simulink model "project_switchcase"  (R2019a)
settings: Solver=FixedStepDiscrete  StartTime=0.0  StopTime=40  FixedStep=1  RelTol=1e-3
libraries: powerlib_meascontrol x10, simulink x1
settings Model: Creator=admin  LastModifiedBy=admin
settings OptimizationCC: DefaultParameterBehavior=Inlined  EnhancedBackFolding=on  PassReuseOutputArgsAs=Individual arguments  OptimizeBlockOrder=speed  DifferentSizesBufferReuse=on  OptimizationCustomize=off
settings DebuggingCC: ParameterTunabilityLossMsg=error
settings SFSimCC: MATLABDynamicMemAlloc=off
settings RTWCC: SystemTargetFile=ert.tlc  TemplateMakefile=ert_default_tmf  GenerateReport=on  IncludeHyperlinkInReport=on  LaunchReport=on  GenerateTraceInfo=on  GenerateTraceReport=on  GenerateTraceReportSl=on  GenerateTraceReportSf=on  GenerateTraceReportEml=on
settings CodeAppCC: ForceParamTrailComments=on  IgnoreCustomStorageClasses=off  OperatorAnnotations=on  SimulinkDataObjDesc=on  SFDataObjDesc=on  InsertBlockDesc=on
settings ERTTargetCC: TargetLangStandard=C99 (ISO)  GenerateSampleERTMain=on  InlinedParameterPlacement=NonHierarchical  ERTCustomFileTemplate=example_file_process.tlc

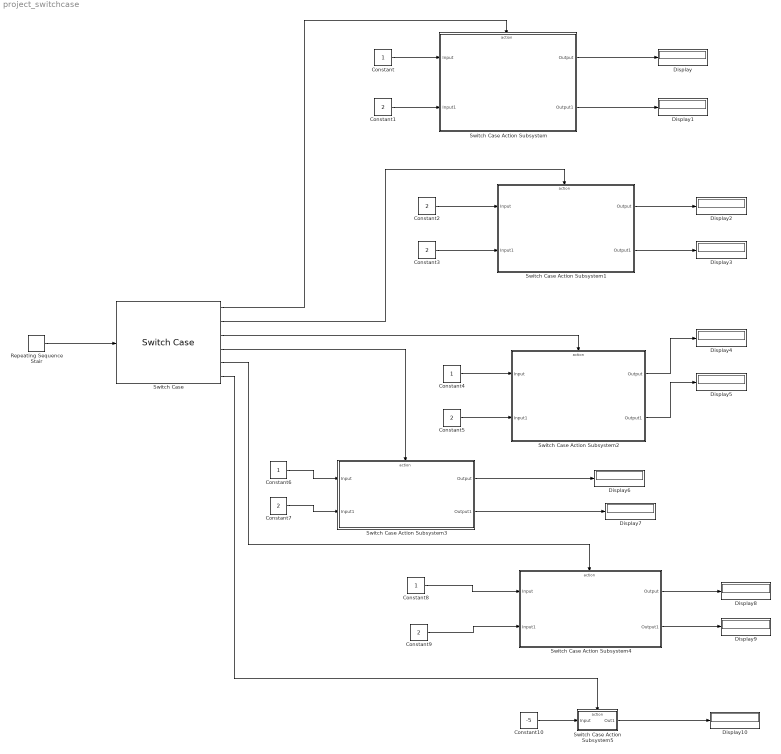
== system project_switchcase ==
  Constant{,4,6,8} (4 alike) : Constant
  Constant{1..3,5,7,9} (6 alike) : Constant  Value=2
  Constant10 : Constant  Value=-5
  Display{,1..10} (11 alike) : Display
  Repeating Sequence Stair : simulink/Sources/Repeating Sequence Stair  OutValues=[1 1 2 2 3 3 4 4 5 5 6 6].'  tsamp=-1  OutMin=[]  OutMax=[]  OutDataTypeStr=double  OutputDataTypeScalingMode=double  OutDataType=fixdt(0,8)  ConRadixGroup=Best Precision: Vector-wise  OutScaling=2^-12
  Switch Case : SwitchCase  CaseConditions={[1 2],[3 4],[5 6],[7 8],[9 10]}
  Switch Case Action Subsystem : Subsystem  TreatAsAtomicUnit=on
  Switch Case Action Subsystem1 : Subsystem  TreatAsAtomicUnit=on
  Switch Case Action Subsystem2 : Subsystem  TreatAsAtomicUnit=on
  Switch Case Action Subsystem3 : Subsystem  TreatAsAtomicUnit=on
  Switch Case Action Subsystem4 : Subsystem  TreatAsAtomicUnit=on
  Switch Case Action Subsystem5 : Subsystem  TreatAsAtomicUnit=on
  wires:
  Switch Case/1 -> Switch Case Action Subsystem/Action
  Switch Case/2 -> Switch Case Action Subsystem1/Action
  Switch Case/3 -> Switch Case Action Subsystem2/Action
  Switch Case/4 -> Switch Case Action Subsystem3/Action
  Switch Case/5 -> Switch Case Action Subsystem4/Action
  Switch Case/6 -> Switch Case Action Subsystem5/Action
  Repeating Sequence Stair/1 -> Switch Case/1
  Switch Case Action Subsystem/1(Output) -> Display/1
  Switch Case Action Subsystem/2(Output1) -> Display1/1
  Switch Case Action Subsystem1/1(Output) -> Display2/1
  Switch Case Action Subsystem1/2(Output1) -> Display3/1
  Switch Case Action Subsystem2/1(Output) -> Display4/1
  Switch Case Action Subsystem2/2(Output1) -> Display5/1
  Switch Case Action Subsystem3/1(Output) -> Display6/1
  Switch Case Action Subsystem3/2(Output1) -> Display7/1
  Switch Case Action Subsystem4/1(Output) -> Display8/1
  Switch Case Action Subsystem4/2(Output1) -> Display9/1
  Switch Case Action Subsystem5/1(Out1) -> Display10/1
  Constant/1 -> Switch Case Action Subsystem/1(Input)
  Constant1/1 -> Switch Case Action Subsystem/2(Input1)
  Constant2/1 -> Switch Case Action Subsystem1/1(Input)
  Constant3/1 -> Switch Case Action Subsystem1/2(Input1)
  Constant4/1 -> Switch Case Action Subsystem2/1(Input)
  Constant5/1 -> Switch Case Action Subsystem2/2(Input1)
  Constant6/1 -> Switch Case Action Subsystem3/1(Input)
  Constant7/1 -> Switch Case Action Subsystem3/2(Input1)
  Constant8/1 -> Switch Case Action Subsystem4/1(Input)
  Constant9/1 -> Switch Case Action Subsystem4/2(Input1)
  Constant10/1 -> Switch Case Action Subsystem5/1(Input)

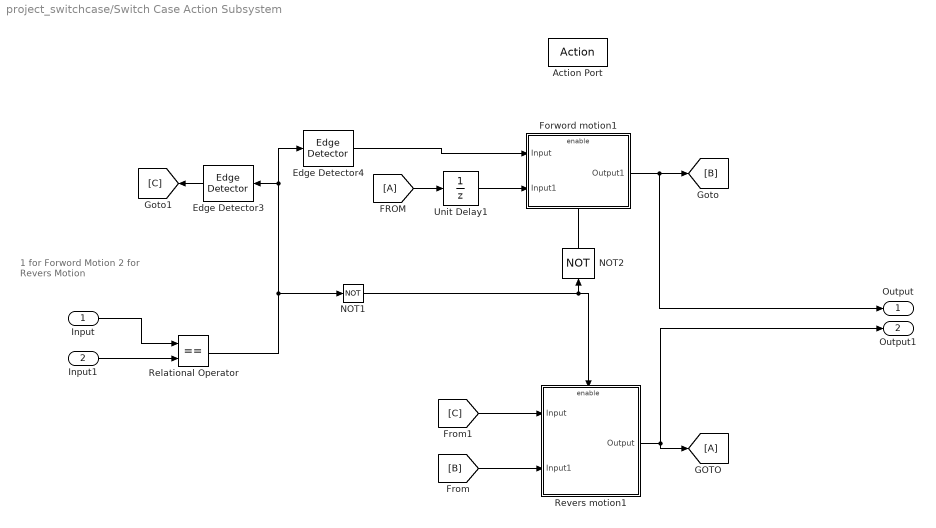
== system project_switchcase/Switch Case Action Subsystem ==
  note: 1 for Forword Motion
      | 2 for Revers Motion
  Input : Inport
  Input1 : Inport  Port=2
  Action Port : ActionPort  ActionPortLabel=case [ 1 2 ]:
  Edge Detector3 : powerlib_meascontrol/Logic/Edge Detector  model=Falling  ic=1  Ts=0
      settings: SourceProductBaseCode=PS
  Edge Detector4 : powerlib_meascontrol/Logic/Edge Detector  model=Rising  ic=1  Ts=0
      settings: SourceProductBaseCode=PS
  Forword motion1 : Subsystem
  NOT1 : Logic  Operator=NOT  IconShape=distinctive  AllPortsSameDT=off  OutDataTypeStr=boolean
  NOT2 : Logic  Operator=NOT  IconShape=distinctive  AllPortsSameDT=off  OutDataTypeStr=boolean
  Relational Operator : RelationalOperator  Operator===  OutDataTypeStr=boolean  RndMeth=Simplest
  Revers motion1 : Subsystem
  Unit Delay1 : UnitDelay  SampleTime=-1  HasFrameUpgradeWarning=on
  Output : Outport
  Output1 : Outport  Port=2
  wires:
  Unit Delay1/1 -> Forword motion1/2(Input1)
  [B] -> Revers motion1/2(Input1)
  Edge Detector4/1 -> Forword motion1/1(Input)
  Revers motion1/1(Output) -> Output1/1, [A]
  Relational Operator/1 -> Edge Detector3/1, Edge Detector4/1, NOT1/1
  Edge Detector3/1 -> [C]
  Input1/1 -> Relational Operator/2
  Input/1 -> Relational Operator/1
  NOT1/1 -> Revers motion1/Enable, NOT2/1
  [A] -> Unit Delay1/1
  NOT2/1 -> Forword motion1/Enable
  [C] -> Revers motion1/1(Input)
  Forword motion1/1(Output1) -> Output/1, [B]

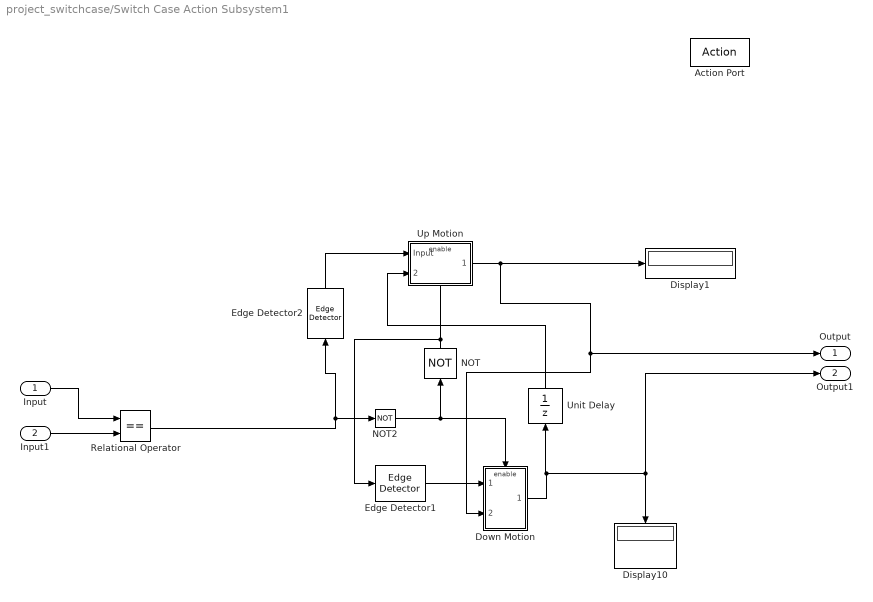
== system project_switchcase/Switch Case Action Subsystem1 ==
  Input : Inport
  Input1 : Inport  Port=2
  Action Port : ActionPort  ActionPortLabel=case [ 3 4 ]:
  Display1 : Display
  Display10 : Display
  Down Motion : Subsystem
  Edge Detector1 : powerlib_meascontrol/Logic/Edge Detector  model=Falling  ic=1  Ts=0
      settings: SourceProductBaseCode=PS
  Edge Detector2 : powerlib_meascontrol/Logic/Edge Detector  model=Rising  ic=1  Ts=0
      settings: SourceProductBaseCode=PS
  NOT : Logic  Operator=NOT  IconShape=distinctive  AllPortsSameDT=off  OutDataTypeStr=boolean
  NOT2 : Logic  Operator=NOT  IconShape=distinctive  AllPortsSameDT=off  OutDataTypeStr=boolean
  Relational Operator : RelationalOperator  Operator===  OutDataTypeStr=boolean  RndMeth=Simplest
  Unit Delay : UnitDelay  SampleTime=-1  HasFrameUpgradeWarning=on
  Up Motion : Subsystem
  Output : Outport
  Output1 : Outport  Port=2
  wires:
  Edge Detector1/1 -> Down Motion/1(Input)
  Down Motion/1(Output) -> Unit Delay/1, Output1/1, Display10/1
  Edge Detector2/1 -> Up Motion/1(Input)
  Up Motion/1(Output1) -> Output/1, Down Motion/2(Input1), Display1/1
  Unit Delay/1 -> Up Motion/2(Input1)
  NOT2/1 -> Down Motion/Enable, NOT/1
  Relational Operator/1 -> Edge Detector2/1, NOT2/1
  Input1/1 -> Relational Operator/2
  NOT/1 -> Edge Detector1/1, Up Motion/Enable
  Input/1 -> Relational Operator/1

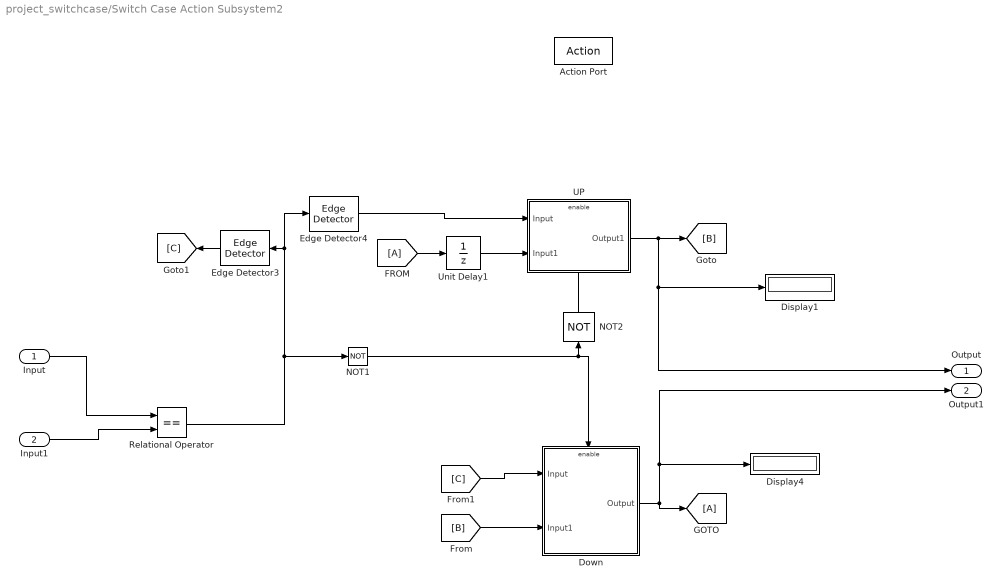
== system project_switchcase/Switch Case Action Subsystem2 ==
  Input : Inport
  Input1 : Inport  Port=2
  Action Port : ActionPort  ActionPortLabel=case [ 5 6 ]:
  Display1 : Display
  Display4 : Display
  Down : Subsystem
  Edge Detector3 : powerlib_meascontrol/Logic/Edge Detector  model=Falling  ic=1  Ts=0
      settings: SourceProductBaseCode=PS
  Edge Detector4 : powerlib_meascontrol/Logic/Edge Detector  model=Rising  ic=1  Ts=0
      settings: SourceProductBaseCode=PS
  NOT1 : Logic  Operator=NOT  IconShape=distinctive  AllPortsSameDT=off  OutDataTypeStr=boolean
  NOT2 : Logic  Operator=NOT  IconShape=distinctive  AllPortsSameDT=off  OutDataTypeStr=boolean
  Relational Operator : RelationalOperator  Operator===  OutDataTypeStr=boolean  RndMeth=Simplest
  UP : Subsystem
  Unit Delay1 : UnitDelay  SampleTime=-1  HasFrameUpgradeWarning=on
  Output : Outport
  Output1 : Outport  Port=2
  wires:
  Edge Detector4/1 -> UP/1(Input)
  [C] -> Down/1(Input)
  [A] -> Unit Delay1/1
  NOT2/1 -> UP/Enable
  Relational Operator/1 -> NOT1/1, Edge Detector4/1, Edge Detector3/1
  Down/1(Output) -> Output1/1, Display4/1, [A]
  Edge Detector3/1 -> [C]
  NOT1/1 -> NOT2/1, Down/Enable
  UP/1(Output1) -> [B], Output/1, Display1/1
  [B] -> Down/2(Input1)
  Unit Delay1/1 -> UP/2(Input1)
  Input/1 -> Relational Operator/1
  Input1/1 -> Relational Operator/2

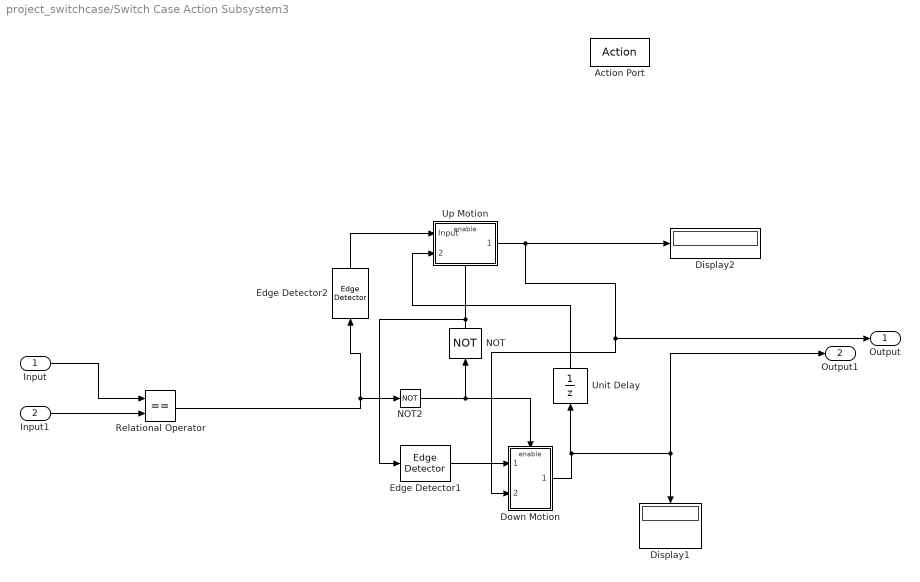
== system project_switchcase/Switch Case Action Subsystem3 ==
  Input : Inport
  Input1 : Inport  Port=2
  Action Port : ActionPort  ActionPortLabel=case [ 7 8 ]:
  Display1 : Display
  Display2 : Display
  Down Motion : Subsystem
  Edge Detector1 : powerlib_meascontrol/Logic/Edge Detector  model=Falling  ic=1  Ts=0
      settings: SourceProductBaseCode=PS
  Edge Detector2 : powerlib_meascontrol/Logic/Edge Detector  model=Rising  ic=1  Ts=0
      settings: SourceProductBaseCode=PS
  NOT : Logic  Operator=NOT  IconShape=distinctive  AllPortsSameDT=off  OutDataTypeStr=boolean
  NOT2 : Logic  Operator=NOT  IconShape=distinctive  AllPortsSameDT=off  OutDataTypeStr=boolean
  Relational Operator : RelationalOperator  Operator===  OutDataTypeStr=boolean  RndMeth=Simplest
  Unit Delay : UnitDelay  SampleTime=-1  HasFrameUpgradeWarning=on
  Up Motion : Subsystem
  Output : Outport
  Output1 : Outport  Port=2
  wires:
  NOT/1 -> Edge Detector1/1, Up Motion/Enable
  Edge Detector1/1 -> Down Motion/1(Input)
  Down Motion/1(Output) -> Unit Delay/1, Output1/1, Display1/1
  Edge Detector2/1 -> Up Motion/1(Input)
  Relational Operator/1 -> Edge Detector2/1, NOT2/1
  Unit Delay/1 -> Up Motion/2(Input1)
  Up Motion/1(Output1) -> Output/1, Down Motion/2(Input1), Display2/1
  NOT2/1 -> Down Motion/Enable, NOT/1
  Input1/1 -> Relational Operator/2
  Input/1 -> Relational Operator/1

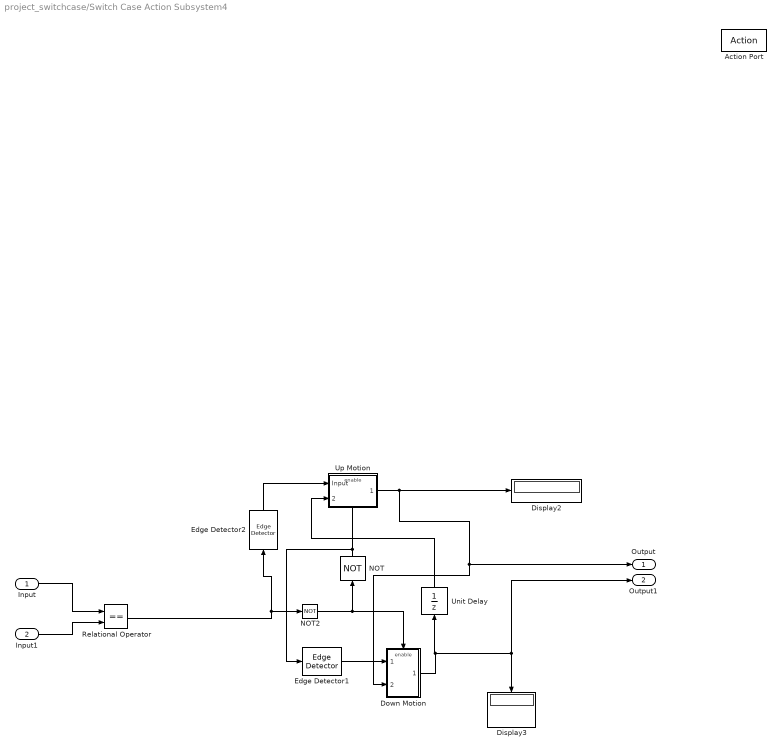
== system project_switchcase/Switch Case Action Subsystem4 ==
  Input : Inport
  Input1 : Inport  Port=2
  Action Port : ActionPort  ActionPortLabel=case [ 9 10 ]:
  Display2 : Display
  Display3 : Display
  Down Motion : Subsystem
  Edge Detector1 : powerlib_meascontrol/Logic/Edge Detector  model=Falling  ic=1  Ts=0
      settings: SourceProductBaseCode=PS
  Edge Detector2 : powerlib_meascontrol/Logic/Edge Detector  model=Rising  ic=1  Ts=0
      settings: SourceProductBaseCode=PS
  NOT : Logic  Operator=NOT  IconShape=distinctive  AllPortsSameDT=off  OutDataTypeStr=boolean
  NOT2 : Logic  Operator=NOT  IconShape=distinctive  AllPortsSameDT=off  OutDataTypeStr=boolean
  Relational Operator : RelationalOperator  Operator===  OutDataTypeStr=boolean  RndMeth=Simplest
  Unit Delay : UnitDelay  SampleTime=-1  HasFrameUpgradeWarning=on
  Up Motion : Subsystem
  Output : Outport
  Output1 : Outport  Port=2
  wires:
  Down Motion/1(Output) -> Unit Delay/1, Output1/1, Display3/1
  Edge Detector2/1 -> Up Motion/1(Input)
  Relational Operator/1 -> Edge Detector2/1, NOT2/1
  Up Motion/1(Output1) -> Output/1, Down Motion/2(Input1), Display2/1
  Edge Detector1/1 -> Down Motion/1(Input)
  NOT/1 -> Edge Detector1/1, Up Motion/Enable
  Unit Delay/1 -> Up Motion/2(Input1)
  NOT2/1 -> Down Motion/Enable, NOT/1
  Input/1 -> Relational Operator/1
  Input1/1 -> Relational Operator/2

== system project_switchcase/Switch Case Action Subsystem5 ==
  Input : Inport
  Action Port : ActionPort  ActionPortLabel=default:
  Out1 : Outport
  wires:
  Input/1 -> Out1/1

== system project_switchcase/Switch Case Action Subsystem/Forword motion1 ==
  Input : Inport
  Input1 : Inport  Port=2
  Enable : EnablePort
  Add1 : Sum
  Constant1 : Constant  Value=100
  Constant2 : Constant  Value=5
  Relational Operator1 : RelationalOperator  Operator=<=  OutDataTypeStr=boolean  RndMeth=Simplest
  Switch1 : Switch  Criteria=u2 ~= 0
  Switch2 : Switch  Criteria=u2 ~= 0
  Unit Delay2 : UnitDelay  SampleTime=-1  HasFrameUpgradeWarning=on
  Output1 : Outport  VectorParamsAs1DForOutWhenUnconnected=on
  wires:
  Constant1/1 -> Switch1/3, Relational Operator1/2
  Relational Operator1/1 -> Switch1/2
  Constant2/1 -> Add1/1
  Add1/1 -> Switch1/1, Relational Operator1/1
  Switch1/1 -> Unit Delay2/1, Output1/1
  Input1/1 -> Switch2/1
  Input/1 -> Switch2/2
  Unit Delay2/1 -> Switch2/3
  Switch2/1 -> Add1/2

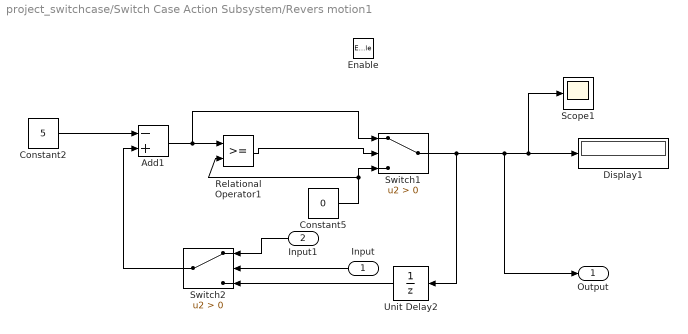
== system project_switchcase/Switch Case Action Subsystem/Revers motion1 ==
  Input : Inport
  Input1 : Inport  Port=2
  Enable : EnablePort
  Add1 : Sum  Inputs=-+
  Constant2 : Constant  Value=5
  Constant5 : Constant  Value=0
  Display1 : Display
  Relational Operator1 : RelationalOperator  OutDataTypeStr=boolean  RndMeth=Simplest
  Scope1 : Scope
  Switch1 : Switch  Criteria=u2 > Threshold
  Switch2 : Switch  Criteria=u2 > Threshold
  Unit Delay2 : UnitDelay  InitialCondition=100  SampleTime=-1  HasFrameUpgradeWarning=on
  Output : Outport  VectorParamsAs1DForOutWhenUnconnected=on
  wires:
  Relational Operator1/1 -> Switch1/2
  Constant2/1 -> Add1/1
  Add1/1 -> Switch1/1, Relational Operator1/1
  Constant5/1 -> Relational Operator1/2, Switch1/3
  Switch1/1 -> Unit Delay2/1, Output/1, Display1/1, Scope1/1
  Switch2/1 -> Add1/2
  Input1/1 -> Switch2/1
  Unit Delay2/1 -> Switch2/3
  Input/1 -> Switch2/2

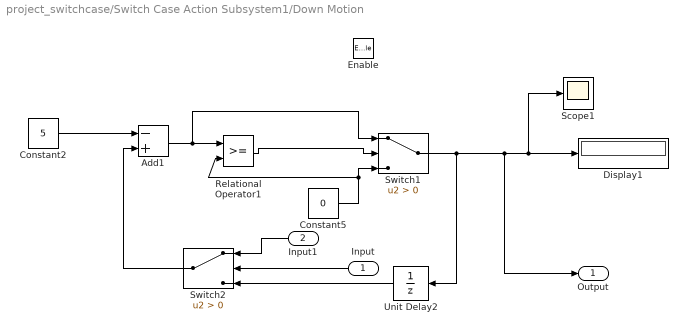
== system project_switchcase/Switch Case Action Subsystem1/Down Motion ==
  Input : Inport
  Input1 : Inport  Port=2
  Enable : EnablePort
  Add1 : Sum  Inputs=-+
  Constant2 : Constant  Value=5
  Constant5 : Constant  Value=0
  Display1 : Display
  Relational Operator1 : RelationalOperator  OutDataTypeStr=boolean  RndMeth=Simplest
  Scope1 : Scope
  Switch1 : Switch  Criteria=u2 > Threshold
  Switch2 : Switch  Criteria=u2 > Threshold
  Unit Delay2 : UnitDelay  InitialCondition=100  SampleTime=-1  HasFrameUpgradeWarning=on
  Output : Outport  VectorParamsAs1DForOutWhenUnconnected=on
  wires:
  Relational Operator1/1 -> Switch1/2
  Constant2/1 -> Add1/1
  Add1/1 -> Switch1/1, Relational Operator1/1
  Constant5/1 -> Relational Operator1/2, Switch1/3
  Switch1/1 -> Unit Delay2/1, Output/1, Display1/1, Scope1/1
  Switch2/1 -> Add1/2
  Input1/1 -> Switch2/1
  Unit Delay2/1 -> Switch2/3
  Input/1 -> Switch2/2

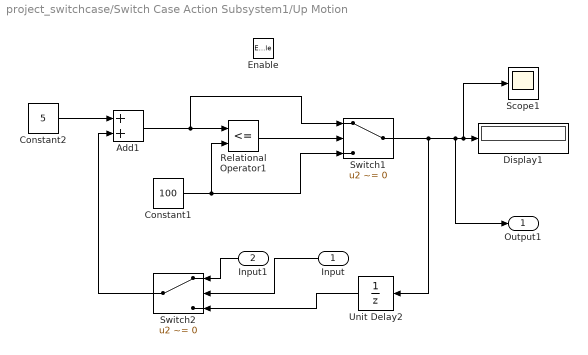
== system project_switchcase/Switch Case Action Subsystem1/Up Motion ==
  Input : Inport
  Input1 : Inport  Port=2
  Enable : EnablePort
  Add1 : Sum
  Constant1 : Constant  Value=100
  Constant2 : Constant  Value=5
  Display1 : Display
  Relational Operator1 : RelationalOperator  Operator=<=  OutDataTypeStr=boolean  RndMeth=Simplest
  Scope1 : Scope
  Switch1 : Switch  Criteria=u2 ~= 0
  Switch2 : Switch  Criteria=u2 ~= 0
  Unit Delay2 : UnitDelay  SampleTime=-1  HasFrameUpgradeWarning=on
  Output1 : Outport  VectorParamsAs1DForOutWhenUnconnected=on
  wires:
  Constant1/1 -> Switch1/3, Relational Operator1/2
  Relational Operator1/1 -> Switch1/2
  Constant2/1 -> Add1/1
  Add1/1 -> Switch1/1, Relational Operator1/1
  Switch1/1 -> Unit Delay2/1, Output1/1, Scope1/1, Display1/1
  Input1/1 -> Switch2/1
  Input/1 -> Switch2/2
  Unit Delay2/1 -> Switch2/3
  Switch2/1 -> Add1/2

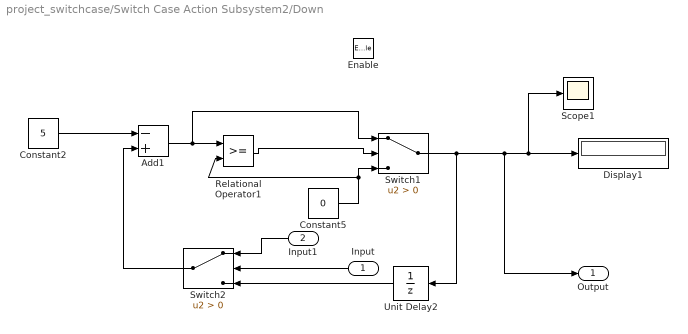
== system project_switchcase/Switch Case Action Subsystem2/Down ==
  Input : Inport
  Input1 : Inport  Port=2
  Enable : EnablePort
  Add1 : Sum  Inputs=-+
  Constant2 : Constant  Value=5
  Constant5 : Constant  Value=0
  Display1 : Display
  Relational Operator1 : RelationalOperator  OutDataTypeStr=boolean  RndMeth=Simplest
  Scope1 : Scope
  Switch1 : Switch  Criteria=u2 > Threshold
  Switch2 : Switch  Criteria=u2 > Threshold
  Unit Delay2 : UnitDelay  InitialCondition=100  SampleTime=-1  HasFrameUpgradeWarning=on
  Output : Outport  VectorParamsAs1DForOutWhenUnconnected=on
  wires:
  Input/1 -> Switch2/2
  Unit Delay2/1 -> Switch2/3
  Input1/1 -> Switch2/1
  Switch2/1 -> Add1/2
  Switch1/1 -> Scope1/1, Display1/1, Output/1, Unit Delay2/1
  Constant5/1 -> Switch1/3, Relational Operator1/2
  Add1/1 -> Relational Operator1/1, Switch1/1
  Constant2/1 -> Add1/1
  Relational Operator1/1 -> Switch1/2

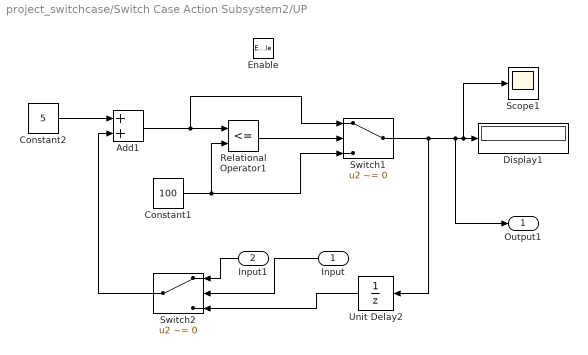
== system project_switchcase/Switch Case Action Subsystem2/UP ==
  Input : Inport
  Input1 : Inport  Port=2
  Enable : EnablePort
  Add1 : Sum
  Constant1 : Constant  Value=100
  Constant2 : Constant  Value=5
  Display1 : Display
  Relational Operator1 : RelationalOperator  Operator=<=  OutDataTypeStr=boolean  RndMeth=Simplest
  Scope1 : Scope
  Switch1 : Switch  Criteria=u2 ~= 0
  Switch2 : Switch  Criteria=u2 ~= 0
  Unit Delay2 : UnitDelay  SampleTime=-1  HasFrameUpgradeWarning=on
  Output1 : Outport  VectorParamsAs1DForOutWhenUnconnected=on
  wires:
  Switch2/1 -> Add1/2
  Unit Delay2/1 -> Switch2/3
  Input/1 -> Switch2/2
  Input1/1 -> Switch2/1
  Switch1/1 -> Display1/1, Scope1/1, Output1/1, Unit Delay2/1
  Add1/1 -> Relational Operator1/1, Switch1/1
  Constant2/1 -> Add1/1
  Relational Operator1/1 -> Switch1/2
  Constant1/1 -> Relational Operator1/2, Switch1/3

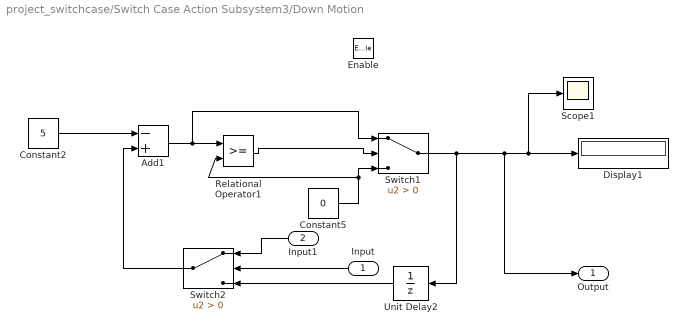
== system project_switchcase/Switch Case Action Subsystem3/Down Motion ==
  Input : Inport
  Input1 : Inport  Port=2
  Enable : EnablePort
  Add1 : Sum  Inputs=-+
  Constant2 : Constant  Value=5
  Constant5 : Constant  Value=0
  Display1 : Display
  Relational Operator1 : RelationalOperator  OutDataTypeStr=boolean  RndMeth=Simplest
  Scope1 : Scope
  Switch1 : Switch  Criteria=u2 > Threshold
  Switch2 : Switch  Criteria=u2 > Threshold
  Unit Delay2 : UnitDelay  InitialCondition=100  SampleTime=-1  HasFrameUpgradeWarning=on
  Output : Outport  VectorParamsAs1DForOutWhenUnconnected=on
  wires:
  Relational Operator1/1 -> Switch1/2
  Constant2/1 -> Add1/1
  Add1/1 -> Switch1/1, Relational Operator1/1
  Constant5/1 -> Relational Operator1/2, Switch1/3
  Switch1/1 -> Unit Delay2/1, Output/1, Display1/1, Scope1/1
  Switch2/1 -> Add1/2
  Input1/1 -> Switch2/1
  Unit Delay2/1 -> Switch2/3
  Input/1 -> Switch2/2

== system project_switchcase/Switch Case Action Subsystem3/Up Motion ==
  Input : Inport
  Input1 : Inport  Port=2
  Enable : EnablePort
  Add1 : Sum
  Constant1 : Constant  Value=100
  Constant2 : Constant  Value=5
  Display1 : Display
  Relational Operator1 : RelationalOperator  Operator=<=  OutDataTypeStr=boolean  RndMeth=Simplest
  Scope1 : Scope
  Switch1 : Switch  Criteria=u2 ~= 0
  Switch2 : Switch  Criteria=u2 ~= 0
  Unit Delay2 : UnitDelay  SampleTime=-1  HasFrameUpgradeWarning=on
  Output1 : Outport  VectorParamsAs1DForOutWhenUnconnected=on
  wires:
  Constant1/1 -> Switch1/3, Relational Operator1/2
  Relational Operator1/1 -> Switch1/2
  Constant2/1 -> Add1/1
  Add1/1 -> Switch1/1, Relational Operator1/1
  Switch1/1 -> Unit Delay2/1, Output1/1, Scope1/1, Display1/1
  Input1/1 -> Switch2/1
  Input/1 -> Switch2/2
  Unit Delay2/1 -> Switch2/3
  Switch2/1 -> Add1/2

== system project_switchcase/Switch Case Action Subsystem4/Down Motion ==
  Input : Inport
  Input1 : Inport  Port=2
  Enable : EnablePort
  Add1 : Sum  Inputs=-+
  Constant2 : Constant  Value=5
  Constant5 : Constant  Value=0
  Display1 : Display
  Relational Operator1 : RelationalOperator  OutDataTypeStr=boolean  RndMeth=Simplest
  Scope1 : Scope
  Switch1 : Switch  Criteria=u2 > Threshold
  Switch2 : Switch  Criteria=u2 > Threshold
  Unit Delay2 : UnitDelay  InitialCondition=100  SampleTime=-1  HasFrameUpgradeWarning=on
  Output : Outport  VectorParamsAs1DForOutWhenUnconnected=on
  wires:
  Relational Operator1/1 -> Switch1/2
  Constant2/1 -> Add1/1
  Add1/1 -> Switch1/1, Relational Operator1/1
  Constant5/1 -> Relational Operator1/2, Switch1/3
  Switch1/1 -> Unit Delay2/1, Output/1, Display1/1, Scope1/1
  Switch2/1 -> Add1/2
  Input1/1 -> Switch2/1
  Unit Delay2/1 -> Switch2/3
  Input/1 -> Switch2/2

== system project_switchcase/Switch Case Action Subsystem4/Up Motion ==
  Input : Inport
  Input1 : Inport  Port=2
  Enable : EnablePort
  Add1 : Sum
  Constant1 : Constant  Value=100
  Constant2 : Constant  Value=5
  Display1 : Display
  Relational Operator1 : RelationalOperator  Operator=<=  OutDataTypeStr=boolean  RndMeth=Simplest
  Scope1 : Scope
  Switch1 : Switch  Criteria=u2 ~= 0
  Switch2 : Switch  Criteria=u2 ~= 0
  Unit Delay2 : UnitDelay  SampleTime=-1  HasFrameUpgradeWarning=on
  Output1 : Outport  VectorParamsAs1DForOutWhenUnconnected=on
  wires:
  Constant1/1 -> Switch1/3, Relational Operator1/2
  Relational Operator1/1 -> Switch1/2
  Constant2/1 -> Add1/1
  Add1/1 -> Switch1/1, Relational Operator1/1
  Switch1/1 -> Unit Delay2/1, Output1/1, Scope1/1, Display1/1
  Input1/1 -> Switch2/1
  Input/1 -> Switch2/2
  Unit Delay2/1 -> Switch2/3
  Switch2/1 -> Add1/2
